simulink model "FSAC2021"  (R2014a)
settings: Solver=FixedStepDiscrete  StartTime=0.0  StopTime=inf  FixedStep=0.0005  RelTol=1e-3
model workspace (MAT data in the model file):
  MCOS : class17 (value not decoded)
  MCOS : class17 (value not decoded)
  MCOS : class17 (value not decoded)
  MCOS : class17 (value not decoded)
  MCOS : class17 (value not decoded)
  MCOS : class17 (value not decoded)
  MCOS : class17 (value not decoded)
  MCOS : class17 (value not decoded)
  MCOS : class17 (value not decoded)
  MCOS : class17 (value not decoded)
  MCOS : class17 (value not decoded)
  MCOS : class17 (value not decoded)
  MCOS : class17 (value not decoded)
  MCOS : class17 (value not decoded)
  MCOS : class17 (value not decoded)
  MCOS : class17 (value not decoded)
  MCOS : class17 (value not decoded)
  MCOS : class17 (value not decoded)
  MCOS : class17 (value not decoded)
  BUZZER_START = 1
  MCOS : class17 (value not decoded)
  MCOS : class17 (value not decoded)
  MCOS : class17 (value not decoded)
  MCOS : class17 (value not decoded)
  MCOS : class17 (value not decoded)
  MCOS : class17 (value not decoded)
  MCOS : class17 (value not decoded)
  MCOS : class17 (value not decoded)
  MCOS : class17 (value not decoded)
  MCOS : class17 (value not decoded)
  MCOS : class17 (value not decoded)
  MCOS : class17 (value not decoded)
  MCOS : class17 (value not decoded)
  MCOS : class17 (value not decoded)
  MCOS : class17 (value not decoded)
  MCOS : class17 (value not decoded)
  MCOS : class17 (value not decoded)
  MCOS : class17 (value not decoded)
  MCOS : class17 (value not decoded)
  MCOS : class17 (value not decoded)
  MCOS : class17 (value not decoded)
  MCOS : class17 (value not decoded)
  MCOS : class17 (value not decoded)
  MCOS : class17 (value not decoded)
  MCOS : class17 (value not decoded)
  MCOS : class17 (value not decoded)
  MCOS : class17 (value not decoded)
  MCOS : class17 (value not decoded)
  MCOS : class17 (value not decoded)
  MCOS : class17 (value not decoded)
  MCOS : class17 (value not decoded)
  MCOS : class17 (value not decoded)
  MCOS : class17 (value not decoded)
  MCOS : class17 (value not decoded)
  MCOS : class17 (value not decoded)
  MCOS : class17 (value not decoded)
  MCOS : class17 (value not decoded)
  MCOS : class17 (value not decoded)
  Brake = 11
  MCOS : class17 (value not decoded)
  MCOS : class17 (value not decoded)
  MCOS : class17 (value not decoded)
  MCOS : class17 (value not decoded)
  MCOS : class17 (value not decoded)
  MCOS : class17 (value not decoded)
  MCOS : class17 (value not decoded)
  MCOS : class17 (value not decoded)
  Sensor_Acc_b = 101.85
  Sensor_Acc_k = -0.0185
  Str_Sen_Orig_Angle = -341
  MCOS : class17 (value not decoded)
  Tire_D = 0.47
  T = 0.05
libraries: simulink x396, ec55xxlib x126
(part 12 of 17)

== system FSAC2021/VCU_CAN_Read/PCANB(BMS、DRIVE_MOTOR)/BMS_HCU_MAXV /BMS_HCU_MAXV ==
  input : Inport
  Demux : Demux  Outputs=8
  MaxCellVoltNo_Ad : Sum
  MaxCellVoltNo_Convert : DataTypeConversion  OutDataTypeStr=uint32
  MaxCellVoltNo_F : Gain
  MaxCellVoltNo_L : simulink/Logic and Bit Operations/Bitwise Operator  logicop=AND  UseBitMask=on  BitMask=255  BitMaskRealWorld=Stored Integer
  MaxCellVoltNo_O : Constant  Value=0  OutDataTypeStr=single
  MaxCellVoltNo_S : ArithShift
  MaxCellVoltNo_Sub : Subsystem
  MaxCellVoltNo_sat : Saturate  UpperLimit=255  LowerLimit=0
  MaxCellVoltNocv : DataTypeConversion
  MaxCellVolt_Ad : Sum
  MaxCellVolt_Convert : DataTypeConversion  OutDataTypeStr=uint32
  MaxCellVolt_F : Gain
  MaxCellVolt_L : simulink/Logic and Bit Operations/Bitwise Operator  logicop=AND  UseBitMask=on  BitMask=65535  BitMaskRealWorld=Stored Integer
  MaxCellVolt_O : Constant  Value=0  OutDataTypeStr=single
  MaxCellVolt_S : ArithShift
  MaxCellVolt_Sub : Subsystem
  MaxCellVolt_sat : Saturate  UpperLimit=5000  LowerLimit=0
  MaxCellVoltcv : DataTypeConversion
  MaxCellVoltinput1_Ad : Sum
  MaxCellVoltinput1_C : Constant  Value=256
  MaxCellVoltinput1_P : Product
  MinCellVoltNo_Ad : Sum
  MinCellVoltNo_Convert : DataTypeConversion  OutDataTypeStr=uint32
  MinCellVoltNo_F : Gain
  MinCellVoltNo_L : simulink/Logic and Bit Operations/Bitwise Operator  logicop=AND  UseBitMask=on  BitMask=255  BitMaskRealWorld=Stored Integer
  MinCellVoltNo_O : Constant  Value=0  OutDataTypeStr=single
  MinCellVoltNo_S : ArithShift
  MinCellVoltNo_Sub : Subsystem
  MinCellVoltNo_sat : Saturate  UpperLimit=255  LowerLimit=0
  MinCellVoltNocv : DataTypeConversion
  MinCellVolt_Ad : Sum
  MinCellVolt_Convert : DataTypeConversion  OutDataTypeStr=uint32
  MinCellVolt_F : Gain
  MinCellVolt_L : simulink/Logic and Bit Operations/Bitwise Operator  logicop=AND  UseBitMask=on  BitMask=65535  BitMaskRealWorld=Stored Integer
  MinCellVolt_O : Constant  Value=0  OutDataTypeStr=single
  MinCellVolt_S : ArithShift
  MinCellVolt_Sub : Subsystem
  MinCellVolt_sat : Saturate  UpperLimit=5000  LowerLimit=0
  MinCellVoltcv : DataTypeConversion
  MinCellVoltinput3_Ad : Sum
  MinCellVoltinput3_C : Constant  Value=256
  MinCellVoltinput3_P : Product
  Terminator : Terminator
  Terminator1 : Terminator
  MaxCellVoltNo_Out : Outport
  MinCellVoltNo_Out : Outport  Port=2
  MinCellVolt_Out : Outport  Port=3
  MaxCellVolt_Out : Outport  Port=4
  wires:
  MaxCellVoltNo_F/1 -> MaxCellVoltNo_Ad/1
  MaxCellVoltNo_O/1 -> MaxCellVoltNo_Ad/2
  MaxCellVoltNo_Ad/1 -> MaxCellVoltNo_sat/1
  MaxCellVoltNo_sat/1 -> MaxCellVoltNo_Out/1
  Demux/6 -> MaxCellVoltNo_Sub/1(In1)
  MaxCellVoltNo_Sub/1(Out1) -> MaxCellVoltNo_Convert/1
  MaxCellVoltNo_Convert/1 -> MaxCellVoltNo_L/1
  MaxCellVoltNo_L/1 -> MaxCellVoltNo_S/1
  MaxCellVoltNo_S/1 -> MaxCellVoltNocv/1
  MaxCellVoltNocv/1 -> MaxCellVoltNo_F/1
  MinCellVoltNo_F/1 -> MinCellVoltNo_Ad/1
  MinCellVoltNo_O/1 -> MinCellVoltNo_Ad/2
  MinCellVoltNo_Ad/1 -> MinCellVoltNo_sat/1
  MinCellVoltNo_sat/1 -> MinCellVoltNo_Out/1
  Demux/5 -> MinCellVoltNo_Sub/1(In1)
  MinCellVoltNo_Sub/1(Out1) -> MinCellVoltNo_Convert/1
  MinCellVoltNo_Convert/1 -> MinCellVoltNo_L/1
  MinCellVoltNo_L/1 -> MinCellVoltNo_S/1
  MinCellVoltNo_S/1 -> MinCellVoltNocv/1
  MinCellVoltNocv/1 -> MinCellVoltNo_F/1
  MinCellVolt_F/1 -> MinCellVolt_Ad/1
  MinCellVolt_O/1 -> MinCellVolt_Ad/2
  MinCellVolt_Ad/1 -> MinCellVolt_sat/1
  MinCellVolt_sat/1 -> MinCellVolt_Out/1
  Demux/3 -> MinCellVoltinput3_P/1
  MinCellVoltinput3_C/1 -> MinCellVoltinput3_P/2
  MinCellVoltinput3_P/1 -> MinCellVoltinput3_Ad/1
  Demux/4 -> MinCellVoltinput3_Ad/2
  MinCellVoltinput3_Ad/1 -> MinCellVolt_Sub/1(In1)
  MinCellVolt_Sub/1(Out1) -> MinCellVolt_Convert/1
  MinCellVolt_Convert/1 -> MinCellVolt_L/1
  MinCellVolt_L/1 -> MinCellVolt_S/1
  MinCellVolt_S/1 -> MinCellVoltcv/1
  MinCellVoltcv/1 -> MinCellVolt_F/1
  MaxCellVolt_F/1 -> MaxCellVolt_Ad/1
  MaxCellVolt_O/1 -> MaxCellVolt_Ad/2
  MaxCellVolt_Ad/1 -> MaxCellVolt_sat/1
  MaxCellVolt_sat/1 -> MaxCellVolt_Out/1
  Demux/1 -> MaxCellVoltinput1_P/1
  MaxCellVoltinput1_C/1 -> MaxCellVoltinput1_P/2
  MaxCellVoltinput1_P/1 -> MaxCellVoltinput1_Ad/1
  Demux/2 -> MaxCellVoltinput1_Ad/2
  MaxCellVoltinput1_Ad/1 -> MaxCellVolt_Sub/1(In1)
  MaxCellVolt_Sub/1(Out1) -> MaxCellVolt_Convert/1
  MaxCellVolt_Convert/1 -> MaxCellVolt_L/1
  MaxCellVolt_L/1 -> MaxCellVolt_S/1
  MaxCellVolt_S/1 -> MaxCellVoltcv/1
  MaxCellVoltcv/1 -> MaxCellVolt_F/1
  input/1 -> Demux/1
  Demux/7 -> Terminator/1
  Demux/8 -> Terminator1/1

== system FSAC2021/VCU_CAN_Read/PCANB(BMS、DRIVE_MOTOR)/BMS_HCU_POWER /BMS_HCU_POWER ==
  input : Inport
  Demux : Demux  Outputs=8
  MaxChrCurtLimit_Ad : Sum
  MaxChrCurtLimit_Convert : DataTypeConversion  OutDataTypeStr=uint32
  MaxChrCurtLimit_F : Gain
  MaxChrCurtLimit_L : simulink/Logic and Bit Operations/Bitwise Operator  logicop=AND  UseBitMask=on  BitMask=65535  BitMaskRealWorld=Stored Integer
  MaxChrCurtLimit_O : Constant  Value=0  OutDataTypeStr=single
  MaxChrCurtLimit_S : ArithShift
  MaxChrCurtLimit_Sub : Subsystem
  MaxChrCurtLimit_sat : Saturate  UpperLimit=1000  LowerLimit=0
  MaxChrCurtLimitcv : DataTypeConversion
  MaxChrCurtLimitinput1_Ad : Sum
  MaxChrCurtLimitinput1_C : Constant  Value=256
  MaxChrCurtLimitinput1_P : Product
  MaxChrPowerLimit_Ad : Sum
  MaxChrPowerLimit_Convert : DataTypeConversion  OutDataTypeStr=uint32
  MaxChrPowerLimit_F : Gain  Gain=0.1
  MaxChrPowerLimit_L : simulink/Logic and Bit Operations/Bitwise Operator  logicop=AND  UseBitMask=on  BitMask=65535  BitMaskRealWorld=Stored Integer
  MaxChrPowerLimit_O : Constant  Value=0  OutDataTypeStr=single
  MaxChrPowerLimit_S : ArithShift
  MaxChrPowerLimit_Sub : Subsystem
  MaxChrPowerLimit_sat : Saturate  UpperLimit=300  LowerLimit=0
  MaxChrPowerLimitcv : DataTypeConversion
  MaxChrPowerLimitinput5_Ad : Sum
  MaxChrPowerLimitinput5_C : Constant  Value=256
  MaxChrPowerLimitinput5_P : Product
  MaxDisCurtLimit_Ad : Sum
  MaxDisCurtLimit_Convert : DataTypeConversion  OutDataTypeStr=uint32
  MaxDisCurtLimit_F : Gain
  MaxDisCurtLimit_L : simulink/Logic and Bit Operations/Bitwise Operator  logicop=AND  UseBitMask=on  BitMask=65535  BitMaskRealWorld=Stored Integer
  MaxDisCurtLimit_O : Constant  Value=0  OutDataTypeStr=single
  MaxDisCurtLimit_S : ArithShift
  MaxDisCurtLimit_Sub : Subsystem
  MaxDisCurtLimit_sat : Saturate  UpperLimit=1000  LowerLimit=0
  MaxDisCurtLimitcv : DataTypeConversion
  MaxDisCurtLimitinput3_Ad : Sum
  MaxDisCurtLimitinput3_C : Constant  Value=256
  MaxDisCurtLimitinput3_P : Product
  MaxDisPowerLimit_Ad : Sum
  MaxDisPowerLimit_Convert : DataTypeConversion  OutDataTypeStr=uint32
  MaxDisPowerLimit_F : Gain  Gain=0.1
  MaxDisPowerLimit_L : simulink/Logic and Bit Operations/Bitwise Operator  logicop=AND  UseBitMask=on  BitMask=65535  BitMaskRealWorld=Stored Integer
  MaxDisPowerLimit_O : Constant  Value=0  OutDataTypeStr=single
  MaxDisPowerLimit_S : ArithShift
  MaxDisPowerLimit_Sub : Subsystem
  MaxDisPowerLimit_sat : Saturate  UpperLimit=300  LowerLimit=0
  MaxDisPowerLimitcv : DataTypeConversion
  MaxDisPowerLimitinput7_Ad : Sum
  MaxDisPowerLimitinput7_C : Constant  Value=256
  MaxDisPowerLimitinput7_P : Product
  MaxDisPowerLimit_Out : Outport
  MaxChrPowerLimit_Out : Outport  Port=2
  MaxDisCurtLimit_Out : Outport  Port=3
  MaxChrCurtLimit_Out : Outport  Port=4
  wires:
  MaxDisPowerLimit_F/1 -> MaxDisPowerLimit_Ad/1
  MaxDisPowerLimit_O/1 -> MaxDisPowerLimit_Ad/2
  MaxDisPowerLimit_Ad/1 -> MaxDisPowerLimit_sat/1
  MaxDisPowerLimit_sat/1 -> MaxDisPowerLimit_Out/1
  Demux/7 -> MaxDisPowerLimitinput7_P/1
  MaxDisPowerLimitinput7_C/1 -> MaxDisPowerLimitinput7_P/2
  MaxDisPowerLimitinput7_P/1 -> MaxDisPowerLimitinput7_Ad/1
  Demux/8 -> MaxDisPowerLimitinput7_Ad/2
  MaxDisPowerLimitinput7_Ad/1 -> MaxDisPowerLimit_Sub/1(In1)
  MaxDisPowerLimit_Sub/1(Out1) -> MaxDisPowerLimit_Convert/1
  MaxDisPowerLimit_Convert/1 -> MaxDisPowerLimit_L/1
  MaxDisPowerLimit_L/1 -> MaxDisPowerLimit_S/1
  MaxDisPowerLimit_S/1 -> MaxDisPowerLimitcv/1
  MaxDisPowerLimitcv/1 -> MaxDisPowerLimit_F/1
  MaxChrPowerLimit_F/1 -> MaxChrPowerLimit_Ad/1
  MaxChrPowerLimit_O/1 -> MaxChrPowerLimit_Ad/2
  MaxChrPowerLimit_Ad/1 -> MaxChrPowerLimit_sat/1
  MaxChrPowerLimit_sat/1 -> MaxChrPowerLimit_Out/1
  Demux/5 -> MaxChrPowerLimitinput5_P/1
  MaxChrPowerLimitinput5_C/1 -> MaxChrPowerLimitinput5_P/2
  MaxChrPowerLimitinput5_P/1 -> MaxChrPowerLimitinput5_Ad/1
  Demux/6 -> MaxChrPowerLimitinput5_Ad/2
  MaxChrPowerLimitinput5_Ad/1 -> MaxChrPowerLimit_Sub/1(In1)
  MaxChrPowerLimit_Sub/1(Out1) -> MaxChrPowerLimit_Convert/1
  MaxChrPowerLimit_Convert/1 -> MaxChrPowerLimit_L/1
  MaxChrPowerLimit_L/1 -> MaxChrPowerLimit_S/1
  MaxChrPowerLimit_S/1 -> MaxChrPowerLimitcv/1
  MaxChrPowerLimitcv/1 -> MaxChrPowerLimit_F/1
  MaxDisCurtLimit_F/1 -> MaxDisCurtLimit_Ad/1
  MaxDisCurtLimit_O/1 -> MaxDisCurtLimit_Ad/2
  MaxDisCurtLimit_Ad/1 -> MaxDisCurtLimit_sat/1
  MaxDisCurtLimit_sat/1 -> MaxDisCurtLimit_Out/1
  Demux/3 -> MaxDisCurtLimitinput3_P/1
  MaxDisCurtLimitinput3_C/1 -> MaxDisCurtLimitinput3_P/2
  MaxDisCurtLimitinput3_P/1 -> MaxDisCurtLimitinput3_Ad/1
  Demux/4 -> MaxDisCurtLimitinput3_Ad/2
  MaxDisCurtLimitinput3_Ad/1 -> MaxDisCurtLimit_Sub/1(In1)
  MaxDisCurtLimit_Sub/1(Out1) -> MaxDisCurtLimit_Convert/1
  MaxDisCurtLimit_Convert/1 -> MaxDisCurtLimit_L/1
  MaxDisCurtLimit_L/1 -> MaxDisCurtLimit_S/1
  MaxDisCurtLimit_S/1 -> MaxDisCurtLimitcv/1
  MaxDisCurtLimitcv/1 -> MaxDisCurtLimit_F/1
  MaxChrCurtLimit_F/1 -> MaxChrCurtLimit_Ad/1
  MaxChrCurtLimit_O/1 -> MaxChrCurtLimit_Ad/2
  MaxChrCurtLimit_Ad/1 -> MaxChrCurtLimit_sat/1
  MaxChrCurtLimit_sat/1 -> MaxChrCurtLimit_Out/1
  Demux/1 -> MaxChrCurtLimitinput1_P/1
  MaxChrCurtLimitinput1_C/1 -> MaxChrCurtLimitinput1_P/2
  MaxChrCurtLimitinput1_P/1 -> MaxChrCurtLimitinput1_Ad/1
  Demux/2 -> MaxChrCurtLimitinput1_Ad/2
  MaxChrCurtLimitinput1_Ad/1 -> MaxChrCurtLimit_Sub/1(In1)
  MaxChrCurtLimit_Sub/1(Out1) -> MaxChrCurtLimit_Convert/1
  MaxChrCurtLimit_Convert/1 -> MaxChrCurtLimit_L/1
  MaxChrCurtLimit_L/1 -> MaxChrCurtLimit_S/1
  MaxChrCurtLimit_S/1 -> MaxChrCurtLimitcv/1
  MaxChrCurtLimitcv/1 -> MaxChrCurtLimit_F/1
  input/1 -> Demux/1

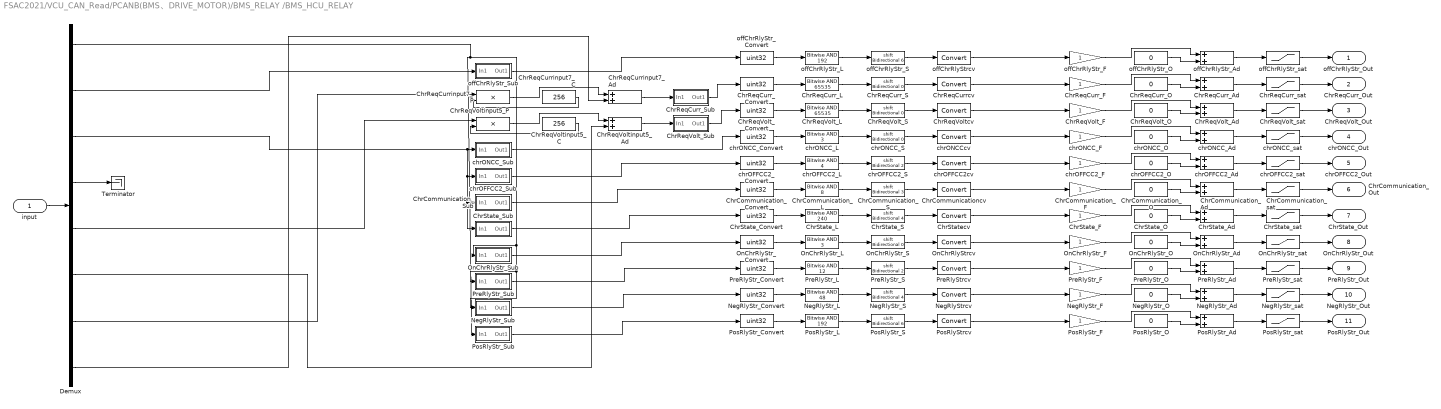
== system FSAC2021/VCU_CAN_Read/PCANB(BMS、DRIVE_MOTOR)/BMS_RELAY /BMS_HCU_RELAY ==
  input : Inport
  ChrCommunication_Ad : Sum
  ChrCommunication_Convert : DataTypeConversion  OutDataTypeStr=uint32
  ChrCommunication_F : Gain
  ChrCommunication_L : simulink/Logic and Bit Operations/Bitwise Operator  logicop=AND  UseBitMask=on  BitMask=8  BitMaskRealWorld=Stored Integer
  ChrCommunication_O : Constant  Value=0  OutDataTypeStr=single
  ChrCommunication_S : ArithShift  BitShiftNumber=3
  ChrCommunication_Sub : Subsystem
  ChrCommunication_sat : Saturate  UpperLimit=1  LowerLimit=0
  ChrCommunicationcv : DataTypeConversion
  ChrReqCurr_Ad : Sum
  ChrReqCurr_Convert : DataTypeConversion  OutDataTypeStr=uint32
  ChrReqCurr_F : Gain
  ChrReqCurr_L : simulink/Logic and Bit Operations/Bitwise Operator  logicop=AND  UseBitMask=on  BitMask=65535  BitMaskRealWorld=Stored Integer
  ChrReqCurr_O : Constant  Value=0  OutDataTypeStr=single
  ChrReqCurr_S : ArithShift
  ChrReqCurr_Sub : Subsystem
  ChrReqCurr_sat : Saturate  UpperLimit=600  LowerLimit=0
  ChrReqCurrcv : DataTypeConversion
  ChrReqCurrinput7_Ad : Sum
  ChrReqCurrinput7_C : Constant  Value=256
  ChrReqCurrinput7_P : Product
  ChrReqVolt_Ad : Sum
  ChrReqVolt_Convert : DataTypeConversion  OutDataTypeStr=uint32
  ChrReqVolt_F : Gain
  ChrReqVolt_L : simulink/Logic and Bit Operations/Bitwise Operator  logicop=AND  UseBitMask=on  BitMask=65535  BitMaskRealWorld=Stored Integer
  ChrReqVolt_O : Constant  Value=0  OutDataTypeStr=single
  ChrReqVolt_S : ArithShift
  ChrReqVolt_Sub : Subsystem
  ChrReqVolt_sat : Saturate  UpperLimit=900  LowerLimit=0
  ChrReqVoltcv : DataTypeConversion
  ChrReqVoltinput5_Ad : Sum
  ChrReqVoltinput5_C : Constant  Value=256
  ChrReqVoltinput5_P : Product
  ChrState_Ad : Sum
  ChrState_Convert : DataTypeConversion  OutDataTypeStr=uint32
  ChrState_F : Gain
  ChrState_L : simulink/Logic and Bit Operations/Bitwise Operator  logicop=AND  UseBitMask=on  BitMask=240  BitMaskRealWorld=Stored Integer
  ChrState_O : Constant  Value=0  OutDataTypeStr=single
  ChrState_S : ArithShift  BitShiftNumber=4
  ChrState_Sub : Subsystem
  ChrState_sat : Saturate  UpperLimit=4  LowerLimit=0
  ChrStatecv : DataTypeConversion
  Demux : Demux  Outputs=8
  NegRlyStr_Ad : Sum
  NegRlyStr_Convert : DataTypeConversion  OutDataTypeStr=uint32
  NegRlyStr_F : Gain
  NegRlyStr_L : simulink/Logic and Bit Operations/Bitwise Operator  logicop=AND  UseBitMask=on  BitMask=48  BitMaskRealWorld=Stored Integer
  NegRlyStr_O : Constant  Value=0  OutDataTypeStr=single
  NegRlyStr_S : ArithShift  BitShiftNumber=4
  NegRlyStr_Sub : Subsystem
  NegRlyStr_sat : Saturate  UpperLimit=2  LowerLimit=0
  NegRlyStrcv : DataTypeConversion
  OnChrRlyStr_Ad : Sum
  OnChrRlyStr_Convert : DataTypeConversion  OutDataTypeStr=uint32
  OnChrRlyStr_F : Gain
  OnChrRlyStr_L : simulink/Logic and Bit Operations/Bitwise Operator  logicop=AND  UseBitMask=on  BitMask=3  BitMaskRealWorld=Stored Integer
  OnChrRlyStr_O : Constant  Value=0  OutDataTypeStr=single
  OnChrRlyStr_S : ArithShift
  OnChrRlyStr_Sub : Subsystem
  OnChrRlyStr_sat : Saturate  UpperLimit=2  LowerLimit=0
  OnChrRlyStrcv : DataTypeConversion
  PosRlyStr_Ad : Sum
  PosRlyStr_Convert : DataTypeConversion  OutDataTypeStr=uint32
  PosRlyStr_F : Gain
  PosRlyStr_L : simulink/Logic and Bit Operations/Bitwise Operator  logicop=AND  UseBitMask=on  BitMask=192  BitMaskRealWorld=Stored Integer
  PosRlyStr_O : Constant  Value=0  OutDataTypeStr=single
  PosRlyStr_S : ArithShift  BitShiftNumber=6
  PosRlyStr_Sub : Subsystem
  PosRlyStr_sat : Saturate  UpperLimit=2  LowerLimit=0
  PosRlyStrcv : DataTypeConversion
  PreRlyStr_Ad : Sum
  PreRlyStr_Convert : DataTypeConversion  OutDataTypeStr=uint32
  PreRlyStr_F : Gain
  PreRlyStr_L : simulink/Logic and Bit Operations/Bitwise Operator  logicop=AND  UseBitMask=on  BitMask=12  BitMaskRealWorld=Stored Integer
  PreRlyStr_O : Constant  Value=0  OutDataTypeStr=single
  PreRlyStr_S : ArithShift  BitShiftNumber=2
  PreRlyStr_Sub : Subsystem
  PreRlyStr_sat : Saturate  UpperLimit=2  LowerLimit=0
  PreRlyStrcv : DataTypeConversion
  Terminator : Terminator
  chrOFFCC2_Ad : Sum
  chrOFFCC2_Convert : DataTypeConversion  OutDataTypeStr=uint32
  chrOFFCC2_F : Gain
  chrOFFCC2_L : simulink/Logic and Bit Operations/Bitwise Operator  logicop=AND  UseBitMask=on  BitMask=4  BitMaskRealWorld=Stored Integer
  chrOFFCC2_O : Constant  Value=0  OutDataTypeStr=single
  chrOFFCC2_S : ArithShift  BitShiftNumber=2
  chrOFFCC2_Sub : Subsystem
  chrOFFCC2_sat : Saturate  UpperLimit=1  LowerLimit=0
  chrOFFCC2cv : DataTypeConversion
  chrONCC_Ad : Sum
  chrONCC_Convert : DataTypeConversion  OutDataTypeStr=uint32
  chrONCC_F : Gain
  chrONCC_L : simulink/Logic and Bit Operations/Bitwise Operator  logicop=AND  UseBitMask=on  BitMask=3  BitMaskRealWorld=Stored Integer
  chrONCC_O : Constant  Value=0  OutDataTypeStr=single
  chrONCC_S : ArithShift
  chrONCC_Sub : Subsystem
  chrONCC_sat : Saturate  UpperLimit=3  LowerLimit=0
  chrONCCcv : DataTypeConversion
  offChrRlyStr_Ad : Sum
  offChrRlyStr_Convert : DataTypeConversion  OutDataTypeStr=uint32
  offChrRlyStr_F : Gain
  offChrRlyStr_L : simulink/Logic and Bit Operations/Bitwise Operator  logicop=AND  UseBitMask=on  BitMask=192  BitMaskRealWorld=Stored Integer
  offChrRlyStr_O : Constant  Value=0  OutDataTypeStr=single
  offChrRlyStr_S : ArithShift  BitShiftNumber=6
  offChrRlyStr_Sub : Subsystem
  offChrRlyStr_sat : Saturate  UpperLimit=2  LowerLimit=0
  offChrRlyStrcv : DataTypeConversion
  offChrRlyStr_Out : Outport
  ChrReqCurr_Out : Outport  Port=2
  ChrReqVolt_Out : Outport  Port=3
  chrONCC_Out : Outport  Port=4
  chrOFFCC2_Out : Outport  Port=5
  ChrCommunication_Out : Outport  Port=6
  ChrState_Out : Outport  Port=7
  OnChrRlyStr_Out : Outport  Port=8
  PreRlyStr_Out : Outport  Port=9
  NegRlyStr_Out : Outport  Port=10
  PosRlyStr_Out : Outport  Port=11
  wires:
  offChrRlyStr_F/1 -> offChrRlyStr_Ad/1
  offChrRlyStr_O/1 -> offChrRlyStr_Ad/2
  offChrRlyStr_Ad/1 -> offChrRlyStr_sat/1
  offChrRlyStr_sat/1 -> offChrRlyStr_Out/1
  Demux/2 -> offChrRlyStr_Sub/1(In1)
  offChrRlyStr_Sub/1(Out1) -> offChrRlyStr_Convert/1
  offChrRlyStr_Convert/1 -> offChrRlyStr_L/1
  offChrRlyStr_L/1 -> offChrRlyStr_S/1
  offChrRlyStr_S/1 -> offChrRlyStrcv/1
  offChrRlyStrcv/1 -> offChrRlyStr_F/1
  ChrReqCurr_F/1 -> ChrReqCurr_Ad/1
  ChrReqCurr_O/1 -> ChrReqCurr_Ad/2
  ChrReqCurr_Ad/1 -> ChrReqCurr_sat/1
  ChrReqCurr_sat/1 -> ChrReqCurr_Out/1
  Demux/7 -> ChrReqCurrinput7_P/1
  ChrReqCurrinput7_C/1 -> ChrReqCurrinput7_P/2
  ChrReqCurrinput7_P/1 -> ChrReqCurrinput7_Ad/1
  Demux/8 -> ChrReqCurrinput7_Ad/2
  ChrReqCurrinput7_Ad/1 -> ChrReqCurr_Sub/1(In1)
  ChrReqCurr_Sub/1(Out1) -> ChrReqCurr_Convert/1
  ChrReqCurr_Convert/1 -> ChrReqCurr_L/1
  ChrReqCurr_L/1 -> ChrReqCurr_S/1
  ChrReqCurr_S/1 -> ChrReqCurrcv/1
  ChrReqCurrcv/1 -> ChrReqCurr_F/1
  ChrReqVolt_F/1 -> ChrReqVolt_Ad/1
  ChrReqVolt_O/1 -> ChrReqVolt_Ad/2
  ChrReqVolt_Ad/1 -> ChrReqVolt_sat/1
  ChrReqVolt_sat/1 -> ChrReqVolt_Out/1
  Demux/5 -> ChrReqVoltinput5_P/1
  ChrReqVoltinput5_C/1 -> ChrReqVoltinput5_P/2
  ChrReqVoltinput5_P/1 -> ChrReqVoltinput5_Ad/1
  Demux/6 -> ChrReqVoltinput5_Ad/2
  ChrReqVoltinput5_Ad/1 -> ChrReqVolt_Sub/1(In1)
  ChrReqVolt_Sub/1(Out1) -> ChrReqVolt_Convert/1
  ChrReqVolt_Convert/1 -> ChrReqVolt_L/1
  ChrReqVolt_L/1 -> ChrReqVolt_S/1
  ChrReqVolt_S/1 -> ChrReqVoltcv/1
  ChrReqVoltcv/1 -> ChrReqVolt_F/1
  chrONCC_F/1 -> chrONCC_Ad/1
  chrONCC_O/1 -> chrONCC_Ad/2
  chrONCC_Ad/1 -> chrONCC_sat/1
  chrONCC_sat/1 -> chrONCC_Out/1
  Demux/3 -> ChrCommunication_Sub/1(In1), ChrState_Sub/1(In1), chrOFFCC2_Sub/1(In1), chrONCC_Sub/1(In1)
  chrONCC_Sub/1(Out1) -> chrONCC_Convert/1
  chrONCC_Convert/1 -> chrONCC_L/1
  chrONCC_L/1 -> chrONCC_S/1
  chrONCC_S/1 -> chrONCCcv/1
  chrONCCcv/1 -> chrONCC_F/1
  chrOFFCC2_F/1 -> chrOFFCC2_Ad/1
  chrOFFCC2_O/1 -> chrOFFCC2_Ad/2
  chrOFFCC2_Ad/1 -> chrOFFCC2_sat/1
  chrOFFCC2_sat/1 -> chrOFFCC2_Out/1
  chrOFFCC2_Sub/1(Out1) -> chrOFFCC2_Convert/1
  chrOFFCC2_Convert/1 -> chrOFFCC2_L/1
  chrOFFCC2_L/1 -> chrOFFCC2_S/1
  chrOFFCC2_S/1 -> chrOFFCC2cv/1
  chrOFFCC2cv/1 -> chrOFFCC2_F/1
  ChrCommunication_F/1 -> ChrCommunication_Ad/1
  ChrCommunication_O/1 -> ChrCommunication_Ad/2
  ChrCommunication_Ad/1 -> ChrCommunication_sat/1
  ChrCommunication_sat/1 -> ChrCommunication_Out/1
  ChrCommunication_Sub/1(Out1) -> ChrCommunication_Convert/1
  ChrCommunication_Convert/1 -> ChrCommunication_L/1
  ChrCommunication_L/1 -> ChrCommunication_S/1
  ChrCommunication_S/1 -> ChrCommunicationcv/1
  ChrCommunicationcv/1 -> ChrCommunication_F/1
  ChrState_F/1 -> ChrState_Ad/1
  ChrState_O/1 -> ChrState_Ad/2
  ChrState_Ad/1 -> ChrState_sat/1
  ChrState_sat/1 -> ChrState_Out/1
  ChrState_Sub/1(Out1) -> ChrState_Convert/1
  ChrState_Convert/1 -> ChrState_L/1
  ChrState_L/1 -> ChrState_S/1
  ChrState_S/1 -> ChrStatecv/1
  ChrStatecv/1 -> ChrState_F/1
  OnChrRlyStr_F/1 -> OnChrRlyStr_Ad/1
  OnChrRlyStr_O/1 -> OnChrRlyStr_Ad/2
  OnChrRlyStr_Ad/1 -> OnChrRlyStr_sat/1
  OnChrRlyStr_sat/1 -> OnChrRlyStr_Out/1
  Demux/1 -> PreRlyStr_Sub/1(In1), NegRlyStr_Sub/1(In1), OnChrRlyStr_Sub/1(In1), PosRlyStr_Sub/1(In1)
  OnChrRlyStr_Sub/1(Out1) -> OnChrRlyStr_Convert/1
  OnChrRlyStr_Convert/1 -> OnChrRlyStr_L/1
  OnChrRlyStr_L/1 -> OnChrRlyStr_S/1
  OnChrRlyStr_S/1 -> OnChrRlyStrcv/1
  OnChrRlyStrcv/1 -> OnChrRlyStr_F/1
  PreRlyStr_F/1 -> PreRlyStr_Ad/1
  PreRlyStr_O/1 -> PreRlyStr_Ad/2
  PreRlyStr_Ad/1 -> PreRlyStr_sat/1
  PreRlyStr_sat/1 -> PreRlyStr_Out/1
  PreRlyStr_Sub/1(Out1) -> PreRlyStr_Convert/1
  PreRlyStr_Convert/1 -> PreRlyStr_L/1
  PreRlyStr_L/1 -> PreRlyStr_S/1
  PreRlyStr_S/1 -> PreRlyStrcv/1
  PreRlyStrcv/1 -> PreRlyStr_F/1
  NegRlyStr_F/1 -> NegRlyStr_Ad/1
  NegRlyStr_O/1 -> NegRlyStr_Ad/2
  NegRlyStr_Ad/1 -> NegRlyStr_sat/1
  NegRlyStr_sat/1 -> NegRlyStr_Out/1
  NegRlyStr_Sub/1(Out1) -> NegRlyStr_Convert/1
  NegRlyStr_Convert/1 -> NegRlyStr_L/1
  NegRlyStr_L/1 -> NegRlyStr_S/1
  NegRlyStr_S/1 -> NegRlyStrcv/1
  NegRlyStrcv/1 -> NegRlyStr_F/1
  PosRlyStr_F/1 -> PosRlyStr_Ad/1
  PosRlyStr_O/1 -> PosRlyStr_Ad/2
  PosRlyStr_Ad/1 -> PosRlyStr_sat/1
  PosRlyStr_sat/1 -> PosRlyStr_Out/1
  PosRlyStr_Sub/1(Out1) -> PosRlyStr_Convert/1
  PosRlyStr_Convert/1 -> PosRlyStr_L/1
  PosRlyStr_L/1 -> PosRlyStr_S/1
  PosRlyStr_S/1 -> PosRlyStrcv/1
  PosRlyStrcv/1 -> PosRlyStr_F/1
  input/1 -> Demux/1
  Demux/4 -> Terminator/1

== system FSAC2021/VCU_CAN_Read/PCANB(BMS、DRIVE_MOTOR)/MOTOR_CURRENT_SPEED/Motor_Currt_Speed_Sub ==
  In1 : Inport
  Out1 : Outport
  wires:
  In1/1 -> Out1/1

== system FSAC2021/VCU_CAN_Read/Subsystem/BMS_HCU_INFO /BMS_HCU_INFO ==
  input : Inport
  BatAlmLv_Ad : Sum
  BatAlmLv_Convert : DataTypeConversion  OutDataTypeStr=uint32
  BatAlmLv_F : Gain
  BatAlmLv_L : simulink/Logic and Bit Operations/Bitwise Operator  logicop=AND  UseBitMask=on  BitMask=15  BitMaskRealWorld=Stored Integer
  BatAlmLv_O : Constant  Value=0  OutDataTypeStr=single
  BatAlmLv_S : ArithShift
  BatAlmLv_Sub : Subsystem
  BatAlmLv_sat : Saturate  UpperLimit=4  LowerLimit=0
  BatAlmLvcv : DataTypeConversion
  BatCurrent_Ad : Sum
  BatCurrent_Convert : DataTypeConversion  OutDataTypeStr=uint32
  BatCurrent_F : Gain  Gain=0.1
  BatCurrent_L : simulink/Logic and Bit Operations/Bitwise Operator  logicop=AND  UseBitMask=on  BitMask=65535  BitMaskRealWorld=Stored Integer
  BatCurrent_O : Constant  Value=-1000  OutDataTypeStr=single
  BatCurrent_S : ArithShift
  BatCurrent_Sub : Subsystem
  BatCurrent_sat : Saturate  UpperLimit=1000  LowerLimit=-1000
  BatCurrentcv : DataTypeConversion
  BatCurrentinput3_Ad : Sum
  BatCurrentinput3_C : Constant  Value=256
  BatCurrentinput3_P : Product
  BatLife_Ad : Sum
  BatLife_Convert : DataTypeConversion  OutDataTypeStr=uint32
  BatLife_F : Gain
  BatLife_L : simulink/Logic and Bit Operations/Bitwise Operator  logicop=AND  UseBitMask=on  BitMask=255  BitMaskRealWorld=Stored Integer
  BatLife_O : Constant  Value=0  OutDataTypeStr=single
  BatLife_S : ArithShift
  BatLife_Sub : Subsystem
  BatLife_sat : Saturate  UpperLimit=255  LowerLimit=0
  BatLifecv : DataTypeConversion
  BatSoc_Ad : Sum
  BatSoc_Convert : DataTypeConversion  OutDataTypeStr=uint32
  BatSoc_F : Gain
  BatSoc_L : simulink/Logic and Bit Operations/Bitwise Operator  logicop=AND  UseBitMask=on  BitMask=255  BitMaskRealWorld=Stored Integer
  BatSoc_O : Constant  Value=0  OutDataTypeStr=single
  BatSoc_S : ArithShift
  BatSoc_Sub : Subsystem
  BatSoc_sat : Saturate  UpperLimit=100  LowerLimit=0
  BatSoccv : DataTypeConversion
  BatSoh_Ad : Sum
  BatSoh_Convert : DataTypeConversion  OutDataTypeStr=uint32
  BatSoh_F : Gain
  BatSoh_L : simulink/Logic and Bit Operations/Bitwise Operator  logicop=AND  UseBitMask=on  BitMask=255  BitMaskRealWorld=Stored Integer
  BatSoh_O : Constant  Value=0  OutDataTypeStr=single
  BatSoh_S : ArithShift
  BatSoh_Sub : Subsystem
  BatSoh_sat : Saturate  UpperLimit=100  LowerLimit=0
  BatSohcv : DataTypeConversion
  BatState_Ad : Sum
  BatState_Convert : DataTypeConversion  OutDataTypeStr=uint32
  BatState_F : Gain
  BatState_L : simulink/Logic and Bit Operations/Bitwise Operator  logicop=AND  UseBitMask=on  BitMask=240  BitMaskRealWorld=Stored Integer
  BatState_O : Constant  Value=0  OutDataTypeStr=single
  BatState_S : ArithShift  BitShiftNumber=4
  BatState_Sub : Subsystem
  BatState_sat : Saturate  UpperLimit=7  LowerLimit=1
  BatStatecv : DataTypeConversion
  BatVoltage_Ad : Sum
  BatVoltage_Convert : DataTypeConversion  OutDataTypeStr=uint32
  BatVoltage_F : Gain  Gain=0.1
  BatVoltage_L : simulink/Logic and Bit Operations/Bitwise Operator  logicop=AND  UseBitMask=on  BitMask=65535  BitMaskRealWorld=Stored Integer
  BatVoltage_O : Constant  Value=0  OutDataTypeStr=single
  BatVoltage_S : ArithShift
  BatVoltage_Sub : Subsystem
  BatVoltage_sat : Saturate  UpperLimit=900  LowerLimit=0
  BatVoltagecv : DataTypeConversion
  BatVoltageinput1_Ad : Sum
  BatVoltageinput1_C : Constant  Value=256
  BatVoltageinput1_P : Product
  Demux : Demux  Outputs=8
  BatLife_Out : Outport
  BatAlmLv_Out : Outport  Port=2
  BatState_Out : Outport  Port=3
  BatSoh_Out : Outport  Port=4
  BatSoc_Out : Outport  Port=5
  BatCurrent_Out : Outport  Port=6
  BatVoltage_Out : Outport  Port=7
  wires:
  BatLife_F/1 -> BatLife_Ad/1
  BatLife_O/1 -> BatLife_Ad/2
  BatLife_Ad/1 -> BatLife_sat/1
  BatLife_sat/1 -> BatLife_Out/1
  Demux/8 -> BatLife_Sub/1(In1)
  BatLife_Sub/1(Out1) -> BatLife_Convert/1
  BatLife_Convert/1 -> BatLife_L/1
  BatLife_L/1 -> BatLife_S/1
  BatLife_S/1 -> BatLifecv/1
  BatLifecv/1 -> BatLife_F/1
  BatAlmLv_F/1 -> BatAlmLv_Ad/1
  BatAlmLv_O/1 -> BatAlmLv_Ad/2
  BatAlmLv_Ad/1 -> BatAlmLv_sat/1
  BatAlmLv_sat/1 -> BatAlmLv_Out/1
  Demux/7 -> BatAlmLv_Sub/1(In1), BatState_Sub/1(In1)
  BatAlmLv_Sub/1(Out1) -> BatAlmLv_Convert/1
  BatAlmLv_Convert/1 -> BatAlmLv_L/1
  BatAlmLv_L/1 -> BatAlmLv_S/1
  BatAlmLv_S/1 -> BatAlmLvcv/1
  BatAlmLvcv/1 -> BatAlmLv_F/1
  BatState_F/1 -> BatState_Ad/1
  BatState_O/1 -> BatState_Ad/2
  BatState_Ad/1 -> BatState_sat/1
  BatState_sat/1 -> BatState_Out/1
  BatState_Sub/1(Out1) -> BatState_Convert/1
  BatState_Convert/1 -> BatState_L/1
  BatState_L/1 -> BatState_S/1
  BatState_S/1 -> BatStatecv/1
  BatStatecv/1 -> BatState_F/1
  BatSoh_F/1 -> BatSoh_Ad/1
  BatSoh_O/1 -> BatSoh_Ad/2
  BatSoh_Ad/1 -> BatSoh_sat/1
  BatSoh_sat/1 -> BatSoh_Out/1
  Demux/6 -> BatSoh_Sub/1(In1)
  BatSoh_Sub/1(Out1) -> BatSoh_Convert/1
  BatSoh_Convert/1 -> BatSoh_L/1
  BatSoh_L/1 -> BatSoh_S/1
  BatSoh_S/1 -> BatSohcv/1
  BatSohcv/1 -> BatSoh_F/1
  BatSoc_F/1 -> BatSoc_Ad/1
  BatSoc_O/1 -> BatSoc_Ad/2
  BatSoc_Ad/1 -> BatSoc_sat/1
  BatSoc_sat/1 -> BatSoc_Out/1
  Demux/5 -> BatSoc_Sub/1(In1)
  BatSoc_Sub/1(Out1) -> BatSoc_Convert/1
  BatSoc_Convert/1 -> BatSoc_L/1
  BatSoc_L/1 -> BatSoc_S/1
  BatSoc_S/1 -> BatSoccv/1
  BatSoccv/1 -> BatSoc_F/1
  BatCurrent_F/1 -> BatCurrent_Ad/1
  BatCurrent_O/1 -> BatCurrent_Ad/2
  BatCurrent_Ad/1 -> BatCurrent_sat/1
  BatCurrent_sat/1 -> BatCurrent_Out/1
  Demux/3 -> BatCurrentinput3_P/1
  BatCurrentinput3_C/1 -> BatCurrentinput3_P/2
  BatCurrentinput3_P/1 -> BatCurrentinput3_Ad/1
  Demux/4 -> BatCurrentinput3_Ad/2
  BatCurrentinput3_Ad/1 -> BatCurrent_Sub/1(In1)
  BatCurrent_Sub/1(Out1) -> BatCurrent_Convert/1
  BatCurrent_Convert/1 -> BatCurrent_L/1
  BatCurrent_L/1 -> BatCurrent_S/1
  BatCurrent_S/1 -> BatCurrentcv/1
  BatCurrentcv/1 -> BatCurrent_F/1
  BatVoltage_F/1 -> BatVoltage_Ad/1
  BatVoltage_O/1 -> BatVoltage_Ad/2
  BatVoltage_Ad/1 -> BatVoltage_sat/1
  BatVoltage_sat/1 -> BatVoltage_Out/1
  Demux/1 -> BatVoltageinput1_P/1
  BatVoltageinput1_C/1 -> BatVoltageinput1_P/2
  BatVoltageinput1_P/1 -> BatVoltageinput1_Ad/1
  Demux/2 -> BatVoltageinput1_Ad/2
  BatVoltageinput1_Ad/1 -> BatVoltage_Sub/1(In1)
  BatVoltage_Sub/1(Out1) -> BatVoltage_Convert/1
  BatVoltage_Convert/1 -> BatVoltage_L/1
  BatVoltage_L/1 -> BatVoltage_S/1
  BatVoltage_S/1 -> BatVoltagecv/1
  BatVoltagecv/1 -> BatVoltage_F/1
  input/1 -> Demux/1

== system FSAC2021/VCU_CAN_Read/Subsystem1/HEARTBEAT /MOTEC_HEARTBEAT ==
  input : Inport
  Demux : Demux  Outputs=1
  Heartbeat_info_Ad : Sum
  Heartbeat_info_Convert : DataTypeConversion  OutDataTypeStr=uint32
  Heartbeat_info_F : Gain
  Heartbeat_info_L : simulink/Logic and Bit Operations/Bitwise Operator  logicop=AND  UseBitMask=on  BitMask=255  BitMaskRealWorld=Stored Integer
  Heartbeat_info_O : Constant  Value=0  OutDataTypeStr=single
  Heartbeat_info_S : ArithShift
  Heartbeat_info_Sub : Subsystem
  Heartbeat_info_sat : Saturate  UpperLimit=255  LowerLimit=0
  Heartbeat_infocv : DataTypeConversion
  Heartbeat_info_Out : Outport
  wires:
  Heartbeat_info_F/1 -> Heartbeat_info_Ad/1
  Heartbeat_info_O/1 -> Heartbeat_info_Ad/2
  Heartbeat_info_Ad/1 -> Heartbeat_info_sat/1
  Heartbeat_info_sat/1 -> Heartbeat_info_Out/1
  Demux/1 -> Heartbeat_info_Sub/1(In1)
  Heartbeat_info_Sub/1(Out1) -> Heartbeat_info_Convert/1
  Heartbeat_info_Convert/1 -> Heartbeat_info_L/1
  Heartbeat_info_L/1 -> Heartbeat_info_S/1
  Heartbeat_info_S/1 -> Heartbeat_infocv/1
  Heartbeat_infocv/1 -> Heartbeat_info_F/1
  input/1 -> Demux/1

== system FSAC2021/VCU_CAN_Read/Subsystem2/MOTEC_STATUS /MOTEC_STATUS ==
  input : Inport
  Demux : Demux  Outputs=2
  Fault_Ad : Sum
  Fault_Convert : DataTypeConversion  OutDataTypeStr=uint32
  Fault_F : Gain
  Fault_L : simulink/Logic and Bit Operations/Bitwise Operator  logicop=AND  UseBitMask=on  BitMask=8  BitMaskRealWorld=Stored Integer
  Fault_O : Constant  Value=0  OutDataTypeStr=single
  Fault_S : ArithShift  BitShiftNumber=3
  Fault_Sub : Subsystem
  Fault_sat : Saturate  UpperLimit=1  LowerLimit=0
  Faultcv : DataTypeConversion
  Operation_Enabled_Ad : Sum
  Operation_Enabled_Convert : DataTypeConversion  OutDataTypeStr=uint32
  Operation_Enabled_F : Gain
  Operation_Enabled_L : simulink/Logic and Bit Operations/Bitwise Operator  logicop=AND  UseBitMask=on  BitMask=4  BitMaskRealWorld=Stored Integer
  Operation_Enabled_O : Constant  Value=0  OutDataTypeStr=single
  Operation_Enabled_S : ArithShift  BitShiftNumber=2
  Operation_Enabled_Sub : Subsystem
  Operation_Enabled_sat : Saturate  UpperLimit=1  LowerLimit=0
  Operation_Enabledcv : DataTypeConversion
  Quick_Stop_Ad : Sum
  Quick_Stop_Convert : DataTypeConversion  OutDataTypeStr=uint32
  Quick_Stop_F : Gain
  Quick_Stop_L : simulink/Logic and Bit Operations/Bitwise Operator  logicop=AND  UseBitMask=on  BitMask=32  BitMaskRealWorld=Stored Integer
  Quick_Stop_O : Constant  Value=0  OutDataTypeStr=single
  Quick_Stop_S : ArithShift  BitShiftNumber=5
  Quick_Stop_Sub : Subsystem
  Quick_Stop_sat : Saturate  UpperLimit=1  LowerLimit=0
  Quick_Stopcv : DataTypeConversion
  Ready_Switch_On_Ad : Sum
  Ready_Switch_On_Convert : DataTypeConversion  OutDataTypeStr=uint32
  Ready_Switch_On_F : Gain
  Ready_Switch_On_L : simulink/Logic and Bit Operations/Bitwise Operator  logicop=AND  UseBitMask=on  BitMask=1  BitMaskRealWorld=Stored Integer
  Ready_Switch_On_O : Constant  Value=0  OutDataTypeStr=single
  Ready_Switch_On_S : ArithShift
  Ready_Switch_On_Sub : Subsystem
  Ready_Switch_On_sat : Saturate  UpperLimit=1  LowerLimit=0
  Ready_Switch_Oncv : DataTypeConversion
  Switch_On_Disabled_Ad : Sum
  Switch_On_Disabled_Convert : DataTypeConversion  OutDataTypeStr=uint32
  Switch_On_Disabled_F : Gain
  Switch_On_Disabled_L : simulink/Logic and Bit Operations/Bitwise Operator  logicop=AND  UseBitMask=on  BitMask=64  BitMaskRealWorld=Stored Integer
  Switch_On_Disabled_O : Constant  Value=0  OutDataTypeStr=single
  Switch_On_Disabled_S : ArithShift  BitShiftNumber=6
  Switch_On_Disabled_Sub : Subsystem
  Switch_On_Disabled_sat : Saturate  UpperLimit=1  LowerLimit=0
  Switch_On_Disabledcv : DataTypeConversion
  Swtiched_On_Ad : Sum
  Swtiched_On_Convert : DataTypeConversion  OutDataTypeStr=uint32
  Swtiched_On_F : Gain
  Swtiched_On_L : simulink/Logic and Bit Operations/Bitwise Operator  logicop=AND  UseBitMask=on  BitMask=2  BitMaskRealWorld=Stored Integer
  Swtiched_On_O : Constant  Value=0  OutDataTypeStr=single
  Swtiched_On_S : ArithShift  BitShiftNumber=1
  Swtiched_On_Sub : Subsystem
  Swtiched_On_sat : Saturate  UpperLimit=1  LowerLimit=0
  Swtiched_Oncv : DataTypeConversion
  Target_Reached_Ad : Sum
  Target_Reached_Convert : DataTypeConversion  OutDataTypeStr=uint32
  Target_Reached_F : Gain
  Target_Reached_L : simulink/Logic and Bit Operations/Bitwise Operator  logicop=AND  UseBitMask=on  BitMask=4  BitMaskRealWorld=Stored Integer
  Target_Reached_O : Constant  Value=0  OutDataTypeStr=single
  Target_Reached_S : ArithShift  BitShiftNumber=2
  Target_Reached_Sub : Subsystem
  Target_Reached_sat : Saturate  UpperLimit=1  LowerLimit=0
  Target_Reachedcv : DataTypeConversion
  Voltage_Enabled_Ad : Sum
  Voltage_Enabled_Convert : DataTypeConversion  OutDataTypeStr=uint32
  Voltage_Enabled_F : Gain
  Voltage_Enabled_L : simulink/Logic and Bit Operations/Bitwise Operator  logicop=AND  UseBitMask=on  BitMask=16  BitMaskRealWorld=Stored Integer
  Voltage_Enabled_O : Constant  Value=0  OutDataTypeStr=single
  Voltage_Enabled_S : ArithShift  BitShiftNumber=4
  Voltage_Enabled_Sub : Subsystem
  Voltage_Enabled_sat : Saturate  UpperLimit=1  LowerLimit=0
  Voltage_Enabledcv : DataTypeConversion
  Warning_Ad : Sum
  Warning_Convert : DataTypeConversion  OutDataTypeStr=uint32
  Warning_F : Gain
  Warning_L : simulink/Logic and Bit Operations/Bitwise Operator  logicop=AND  UseBitMask=on  BitMask=128  BitMaskRealWorld=Stored Integer
  Warning_O : Constant  Value=0  OutDataTypeStr=single
  Warning_S : ArithShift  BitShiftNumber=7
  Warning_Sub : Subsystem
  Warning_sat : Saturate  UpperLimit=1  LowerLimit=0
  Warningcv : DataTypeConversion
  Fault_Out : Outport
  Operation_Enabled_Out : Outport  Port=2
  Quick_Stop_Out : Outport  Port=3
  Ready_Switch_On_Out : Outport  Port=4
  Switch_On_Disabled_Out : Outport  Port=5
  Swtiched_On_Out : Outport  Port=6
  Target_Reached_Out : Outport  Port=7
  Voltage_Enabled_Out : Outport  Port=8
  Warning_Out : Outport  Port=9
  wires:
  Fault_F/1 -> Fault_Ad/1
  Fault_O/1 -> Fault_Ad/2
  Fault_Ad/1 -> Fault_sat/1
  Fault_sat/1 -> Fault_Out/1
  Demux/1 -> Swtiched_On_Sub/1(In1), Voltage_Enabled_Sub/1(In1), Switch_On_Disabled_Sub/1(In1), Ready_Switch_On_Sub/1(In1), Quick_Stop_Sub/1(In1), Operation_Enabled_Sub/1(In1), Warning_Sub/1(In1), Fault_Sub/1(In1)
  Fault_Sub/1(Out1) -> Fault_Convert/1
  Fault_Convert/1 -> Fault_L/1
  Fault_L/1 -> Fault_S/1
  Fault_S/1 -> Faultcv/1
  Faultcv/1 -> Fault_F/1
  Operation_Enabled_F/1 -> Operation_Enabled_Ad/1
  Operation_Enabled_O/1 -> Operation_Enabled_Ad/2
  Operation_Enabled_Ad/1 -> Operation_Enabled_sat/1
  Operation_Enabled_sat/1 -> Operation_Enabled_Out/1
  Operation_Enabled_Sub/1(Out1) -> Operation_Enabled_Convert/1
  Operation_Enabled_Convert/1 -> Operation_Enabled_L/1
  Operation_Enabled_L/1 -> Operation_Enabled_S/1
  Operation_Enabled_S/1 -> Operation_Enabledcv/1
  Operation_Enabledcv/1 -> Operation_Enabled_F/1
  Quick_Stop_F/1 -> Quick_Stop_Ad/1
  Quick_Stop_O/1 -> Quick_Stop_Ad/2
  Quick_Stop_Ad/1 -> Quick_Stop_sat/1
  Quick_Stop_sat/1 -> Quick_Stop_Out/1
  Quick_Stop_Sub/1(Out1) -> Quick_Stop_Convert/1
  Quick_Stop_Convert/1 -> Quick_Stop_L/1
  Quick_Stop_L/1 -> Quick_Stop_S/1
  Quick_Stop_S/1 -> Quick_Stopcv/1
  Quick_Stopcv/1 -> Quick_Stop_F/1
  Ready_Switch_On_F/1 -> Ready_Switch_On_Ad/1
  Ready_Switch_On_O/1 -> Ready_Switch_On_Ad/2
  Ready_Switch_On_Ad/1 -> Ready_Switch_On_sat/1
  Ready_Switch_On_sat/1 -> Ready_Switch_On_Out/1
  Ready_Switch_On_Sub/1(Out1) -> Ready_Switch_On_Convert/1
  Ready_Switch_On_Convert/1 -> Ready_Switch_On_L/1
  Ready_Switch_On_L/1 -> Ready_Switch_On_S/1
  Ready_Switch_On_S/1 -> Ready_Switch_Oncv/1
  Ready_Switch_Oncv/1 -> Ready_Switch_On_F/1
  Switch_On_Disabled_F/1 -> Switch_On_Disabled_Ad/1
  Switch_On_Disabled_O/1 -> Switch_On_Disabled_Ad/2
  Switch_On_Disabled_Ad/1 -> Switch_On_Disabled_sat/1
  Switch_On_Disabled_sat/1 -> Switch_On_Disabled_Out/1
  Switch_On_Disabled_Sub/1(Out1) -> Switch_On_Disabled_Convert/1
  Switch_On_Disabled_Convert/1 -> Switch_On_Disabled_L/1
  Switch_On_Disabled_L/1 -> Switch_On_Disabled_S/1
  Switch_On_Disabled_S/1 -> Switch_On_Disabledcv/1
  Switch_On_Disabledcv/1 -> Switch_On_Disabled_F/1
  Swtiched_On_F/1 -> Swtiched_On_Ad/1
  Swtiched_On_O/1 -> Swtiched_On_Ad/2
  Swtiched_On_Ad/1 -> Swtiched_On_sat/1
  Swtiched_On_sat/1 -> Swtiched_On_Out/1
  Swtiched_On_Sub/1(Out1) -> Swtiched_On_Convert/1
  Swtiched_On_Convert/1 -> Swtiched_On_L/1
  Swtiched_On_L/1 -> Swtiched_On_S/1
  Swtiched_On_S/1 -> Swtiched_Oncv/1
  Swtiched_Oncv/1 -> Swtiched_On_F/1
  Target_Reached_F/1 -> Target_Reached_Ad/1
  Target_Reached_O/1 -> Target_Reached_Ad/2
  Target_Reached_Ad/1 -> Target_Reached_sat/1
  Target_Reached_sat/1 -> Target_Reached_Out/1
  Demux/2 -> Target_Reached_Sub/1(In1)
  Target_Reached_Sub/1(Out1) -> Target_Reached_Convert/1
  Target_Reached_Convert/1 -> Target_Reached_L/1
  Target_Reached_L/1 -> Target_Reached_S/1
  Target_Reached_S/1 -> Target_Reachedcv/1
  Target_Reachedcv/1 -> Target_Reached_F/1
  Voltage_Enabled_F/1 -> Voltage_Enabled_Ad/1
  Voltage_Enabled_O/1 -> Voltage_Enabled_Ad/2
  Voltage_Enabled_Ad/1 -> Voltage_Enabled_sat/1
  Voltage_Enabled_sat/1 -> Voltage_Enabled_Out/1
  Voltage_Enabled_Sub/1(Out1) -> Voltage_Enabled_Convert/1
  Voltage_Enabled_Convert/1 -> Voltage_Enabled_L/1
  Voltage_Enabled_L/1 -> Voltage_Enabled_S/1
  Voltage_Enabled_S/1 -> Voltage_Enabledcv/1
  Voltage_Enabledcv/1 -> Voltage_Enabled_F/1
  Warning_F/1 -> Warning_Ad/1
  Warning_O/1 -> Warning_Ad/2
  Warning_Ad/1 -> Warning_sat/1
  Warning_sat/1 -> Warning_Out/1
  Warning_Sub/1(Out1) -> Warning_Convert/1
  Warning_Convert/1 -> Warning_L/1
  Warning_L/1 -> Warning_S/1
  Warning_S/1 -> Warningcv/1
  Warningcv/1 -> Warning_F/1
  input/1 -> Demux/1

== system FSAC2021/Controller/BCU_Controller/Brk_Move/Enabled Subsystem/Angle2Pulses ==
  Angle : Inport
  Angle2Circle : Gain  Gain=-0.0028  OutDataTypeStr=single
  CircleTrans : Gain  Gain=BRK_MTR_RATIO  ParamDataTypeStr=uint8  OutDataTypeStr=int16
  Gain : Gain  Gain=PULSES_PER_CIRCLE  ParamDataTypeStr=uint16  OutDataTypeStr=int16
  Pulses : Outport
  wires:
  Gain/1 -> Pulses/1
  Angle2Circle/1 -> CircleTrans/1
  CircleTrans/1 -> Gain/1
  Angle/1 -> Angle2Circle/1

== system FSAC2021/Controller/BCU_Controller/Brk_Move/Enabled Subsystem1/Angle2Pulses ==
  Angle : Inport
  Angle2Circle : Gain  Gain=0.0028  OutDataTypeStr=single
  CircleTrans : Gain  Gain=BRK_MTR_RATIO  ParamDataTypeStr=uint8  OutDataTypeStr=int16
  Gain : Gain  Gain=PULSES_PER_CIRCLE  ParamDataTypeStr=uint16  OutDataTypeStr=int16
  Pulses : Outport
  wires:
  Gain/1 -> Pulses/1
  Angle2Circle/1 -> CircleTrans/1
  CircleTrans/1 -> Gain/1
  Angle/1 -> Angle2Circle/1

== system FSAC2021/Controller/BCU_Controller/Brk_Move/Enabled Subsystem2/Angle2Pulses ==
  Angle : Inport
  Angle2Circle : Gain  Gain=0.0028  OutDataTypeStr=single
  CircleTrans : Gain  Gain=BRK_MTR_RATIO  ParamDataTypeStr=uint8  OutDataTypeStr=single
  Gain : Gain  Gain=PULSES_PER_CIRCLE  ParamDataTypeStr=uint16  OutDataTypeStr=int16
  Pulses : Outport
  wires:
  Gain/1 -> Pulses/1
  Angle2Circle/1 -> CircleTrans/1
  CircleTrans/1 -> Gain/1
  Angle/1 -> Angle2Circle/1

== system FSAC2021/Input_Process/KL_Sig_Process/Whl_Spd_Process/Whl2Veh_Spd_Trans/Round ==
  Origin_Precision : Inport
  Gain1 : Gain  Gain=10  ParamDataTypeStr=uint8  OutDataTypeStr=uint8  RndMeth=Round
  Gain2 : Gain  Gain=0.1  ParamDataTypeStr=single  OutDataTypeStr=single
  Two_Precision : Outport
  wires:
  Gain2/1 -> Two_Precision/1
  Gain1/1 -> Gain2/1
  Origin_Precision/1 -> Gain1/1

== system FSAC2021/Input_Process/KL_Sig_Process/Whl_Spd_Process/Whl2Veh_Spd_Trans/Wheel_Mean ==
  Wheel_speed_rightrear_wheel : Inport
  Wheel_speed_right_front_wheel : Inport  Port=2
  Wheel_speed_leftrear_wheel : Inport  Port=3
  Wheel_speed_leftfront_wheel : Inport  Port=4
  Add3 : Sum  Inputs=++++
  Gain6 : Gain  Gain=0.25  ParamDataTypeStr=single
  Out1 : Outport
  wires:
  Wheel_speed_leftfront_wheel/1 -> Add3/4
  Wheel_speed_rightrear_wheel/1 -> Add3/1
  Wheel_speed_leftrear_wheel/1 -> Add3/3
  Wheel_speed_right_front_wheel/1 -> Add3/2
  Add3/1 -> Gain6/1
  Gain6/1 -> Out1/1

== system FSAC2021/Input_Process/KL_Sig_Process/Whl_Spd_Process/Whl2Veh_Spd_Trans/rpm2km_h ==
  rpm : Inport
  Gain : Gain  Gain=2*pi*Tire_Radius*3.6/60000
  kmph : Outport
  wires:
  Gain/1 -> kmph/1
  rpm/1 -> Gain/1

== system FSAC2021/ROUTING/TO_DCAN/Subsystem/DIAG_BCU/Brake_0rigin_End_flag ==
  Brake_0rigin_End_flag : Inport
  Brake_0rigin_End_flagRon : Rounding  Operator=round
  Brake_0rigin_End_flag_1sat : Saturate  UpperLimit=4  LowerLimit=0
  Brake_0rigin_End_flag_Convert : DataTypeConversion  OutDataTypeStr=uint8
  Brake_0rigin_End_flag_Convert1 : DataTypeConversion  OutDataTypeStr=uint32
  Brake_0rigin_End_flag_D : Product  Inputs=*/
  Brake_0rigin_End_flag_F : Constant  OutDataTypeStr=single
  Brake_0rigin_End_flag_L : simulink/Logic and Bit Operations/Bitwise Operator  logicop=AND  UseBitMask=on  BitMask=4  BitMaskRealWorld=Stored Integer
  Brake_0rigin_End_flag_O : Constant  Value=0  OutDataTypeStr=single
  Brake_0rigin_End_flag_S : ArithShift  BitShiftNumber=-2
  Brake_0rigin_End_flag_sat : Saturate  UpperLimit=1  LowerLimit=0
  Brake_0rigin_End_flag_st : Sum  Inputs=+-
  output4 : Outport
  wires:
  Brake_0rigin_End_flag/1 -> Brake_0rigin_End_flag_sat/1
  Brake_0rigin_End_flag_sat/1 -> Brake_0rigin_End_flag_st/1
  Brake_0rigin_End_flag_O/1 -> Brake_0rigin_End_flag_st/2
  Brake_0rigin_End_flag_st/1 -> Brake_0rigin_End_flag_D/1
  Brake_0rigin_End_flag_F/1 -> Brake_0rigin_End_flag_D/2
  Brake_0rigin_End_flag_D/1 -> Brake_0rigin_End_flagRon/1
  Brake_0rigin_End_flagRon/1 -> Brake_0rigin_End_flag_S/1
  Brake_0rigin_End_flag_S/1 -> Brake_0rigin_End_flag_1sat/1
  Brake_0rigin_End_flag_1sat/1 -> Brake_0rigin_End_flag_Convert1/1
  Brake_0rigin_End_flag_Convert1/1 -> Brake_0rigin_End_flag_L/1
  Brake_0rigin_End_flag_L/1 -> Brake_0rigin_End_flag_Convert/1
  Brake_0rigin_End_flag_Convert/1 -> output4/1

== system FSAC2021/ROUTING/TO_DCAN/Subsystem/DIAG_BCU/Brake_Current_Position ==
  Brake_Current_Position : Inport
  Brake_Current_PositionBitCov : DataTypeConversion  OutDataTypeStr=uint8
  Brake_Current_PositionCOV : DataTypeConversion  OutDataTypeStr=uint8
  Brake_Current_PositionRon : Rounding  Operator=round
  Brake_Current_Position_1sat : Saturate  UpperLimit=65535  LowerLimit=0
  Brake_Current_Position_And : simulink/Logic and Bit Operations/Bitwise Operator  logicop=AND  UseBitMask=off  NumInputPorts=2  BitMask=bin2dec('11011001')  BitMaskRealWorld=Stored Integer
  Brake_Current_Position_And_C : Constant  Value=255  OutDataTypeStr=uint32
  Brake_Current_Position_Convert : DataTypeConversion  OutDataTypeStr=uint32
  Brake_Current_Position_D : Product  Inputs=*/
  Brake_Current_Position_D1 : Product  Inputs=*/
  Brake_Current_Position_F : Constant  OutDataTypeStr=single
  Brake_Current_Position_L : simulink/Logic and Bit Operations/Bitwise Operator  logicop=AND  UseBitMask=on  BitMask=65535  BitMaskRealWorld=Stored Integer
  Brake_Current_Position_O : Constant  Value=0  OutDataTypeStr=single
  Brake_Current_Position_S : ArithShift
  Brake_Current_Position_sat : Saturate  UpperLimit=65535  LowerLimit=0
  Brake_Current_Position_st : Sum  Inputs=+-
  Brake_Current_Positionoutput1_C : Constant  Value=256
  output1 : Outport
  output2 : Outport  Port=2
  wires:
  Brake_Current_Position/1 -> Brake_Current_Position_sat/1
  Brake_Current_Position_sat/1 -> Brake_Current_Position_st/1
  Brake_Current_Position_O/1 -> Brake_Current_Position_st/2
  Brake_Current_Position_st/1 -> Brake_Current_Position_D/1
  Brake_Current_Position_F/1 -> Brake_Current_Position_D/2
  Brake_Current_Position_D/1 -> Brake_Current_PositionRon/1
  Brake_Current_PositionRon/1 -> Brake_Current_Position_S/1
  Brake_Current_Position_S/1 -> Brake_Current_Position_1sat/1
  Brake_Current_Position_1sat/1 -> Brake_Current_Position_Convert/1
  Brake_Current_Position_Convert/1 -> Brake_Current_Position_L/1
  Brake_Current_Position_L/1 -> Brake_Current_Position_D1/1, Brake_Current_Position_And/1
  Brake_Current_Positionoutput1_C/1 -> Brake_Current_Position_D1/2
  Brake_Current_Position_D1/1 -> Brake_Current_PositionCOV/1
  Brake_Current_PositionCOV/1 -> output1/1
  Brake_Current_Position_And_C/1 -> Brake_Current_Position_And/2
  Brake_Current_Position_And/1 -> Brake_Current_PositionBitCov/1
  Brake_Current_PositionBitCov/1 -> output2/1

== system FSAC2021/ROUTING/TO_DCAN/Subsystem/DIAG_BCU/Brake_cmd_fault_flag ==
  Brake_cmd_fault_flag : Inport
  Brake_cmd_fault_flagRon : Rounding  Operator=round
  Brake_cmd_fault_flag_1sat : Saturate  UpperLimit=128  LowerLimit=0
  Brake_cmd_fault_flag_Convert : DataTypeConversion  OutDataTypeStr=uint8
  Brake_cmd_fault_flag_Convert1 : DataTypeConversion  OutDataTypeStr=uint32
  Brake_cmd_fault_flag_D : Product  Inputs=*/
  Brake_cmd_fault_flag_F : Constant  OutDataTypeStr=single
  Brake_cmd_fault_flag_L : simulink/Logic and Bit Operations/Bitwise Operator  logicop=AND  UseBitMask=on  BitMask=128  BitMaskRealWorld=Stored Integer
  Brake_cmd_fault_flag_O : Constant  Value=0  OutDataTypeStr=single
  Brake_cmd_fault_flag_S : ArithShift  BitShiftNumber=-7
  Brake_cmd_fault_flag_sat : Saturate  UpperLimit=0  LowerLimit=0
  Brake_cmd_fault_flag_st : Sum  Inputs=+-
  output4 : Outport
  wires:
  Brake_cmd_fault_flag/1 -> Brake_cmd_fault_flag_sat/1
  Brake_cmd_fault_flag_sat/1 -> Brake_cmd_fault_flag_st/1
  Brake_cmd_fault_flag_O/1 -> Brake_cmd_fault_flag_st/2
  Brake_cmd_fault_flag_st/1 -> Brake_cmd_fault_flag_D/1
  Brake_cmd_fault_flag_F/1 -> Brake_cmd_fault_flag_D/2
  Brake_cmd_fault_flag_D/1 -> Brake_cmd_fault_flagRon/1
  Brake_cmd_fault_flagRon/1 -> Brake_cmd_fault_flag_S/1
  Brake_cmd_fault_flag_S/1 -> Brake_cmd_fault_flag_1sat/1
  Brake_cmd_fault_flag_1sat/1 -> Brake_cmd_fault_flag_Convert1/1
  Brake_cmd_fault_flag_Convert1/1 -> Brake_cmd_fault_flag_L/1
  Brake_cmd_fault_flag_L/1 -> Brake_cmd_fault_flag_Convert/1
  Brake_cmd_fault_flag_Convert/1 -> output4/1
